simulink library "posAug_cl_old"  (R2022a)
settings: Solver=VariableStepAuto  StartTime=0.0  StopTime=10.0  RelTol=1e-3
undefined symbols (not defined in the file): aoaStart, elevSet, elevStart, env, FLIGHTCONTROLLER, fltCtrl, initializeBussesFromBlock, intSat, pathLaps, pathLapsYaw, posAug, rollAmp, rollFreq, rollPhase, sEstim, slfExitTime, thetaIGain, thetaPGain, vhcl, yawAmp, yawFreq, yawPhase
libraries: slpidlib x10, simulink x5, posAug_cl_new x4, velocityAngle_ul x4, dspsigops x3, pathFollowingCtrlAoATurb_cl x1, pathFollowingCtrlAoATurbCoef_cl x1, courseFollowLookAhead_cl x1, ctrlAllocMatrix3CompCoef_cl x1, eulAng2RotMat_ul x1, $bdroot x1, angleBtw2Vecs_ul x1
(part 2 of 3)

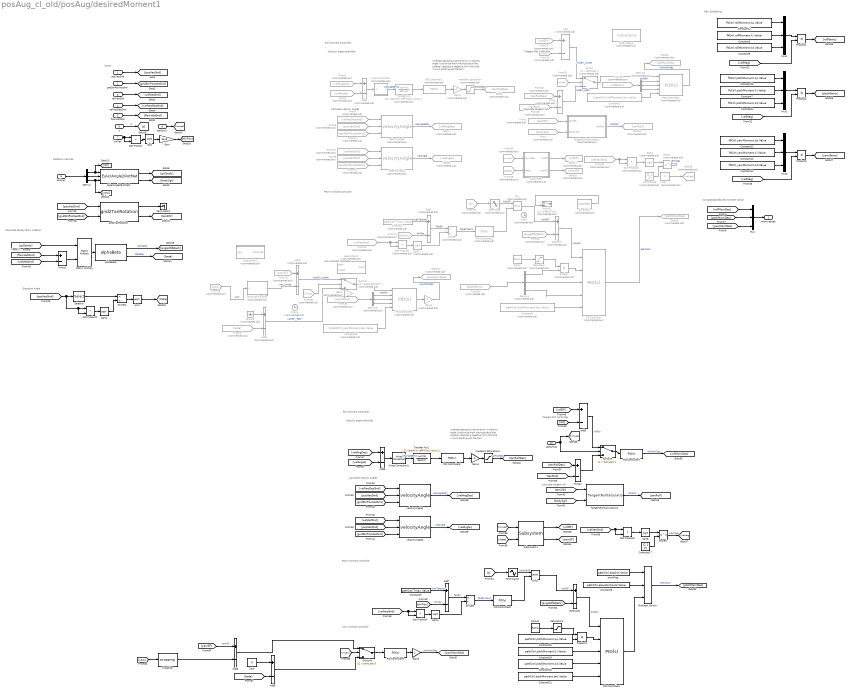
== system posAug_cl_old/posAug/desiredMoment1 ==
  note: Elevation Angle
  note: Yaw moment controller
  note: Pitch moment controller
  note: Inverted because a potive error
      | in velocity angle (clockwise from the
      | outside of the sphere) requires a negative
      | roll (With the X-Axis pointing out the tail)
  note: Velocity angle controller
  note: Inputs
  note: Rotation matrices
  note: Calculate velocity angles
  note: Calculate tangent roll
  note: Tangent Roll Controller
  note: Concatenate desired moment vector
  note: Calculate aerodynamic sideslip
  note: Roll Moment Controller
  note: Gain Scheduling
  note: Inverted because a potive error
      | in velocity angle (clockwise from the
      | outside of the sphere) requires a negative
      | roll (With the X-Axis pointing out the tail)
  note: Velocity angle controller
  note: Calculate tangent roll
  note: Calculate velocity angles
  note: Yaw moment controller
  note: Pitch moment controller
  note: Tangent Roll Controller
  note: Roll Moment Controller
  posVecGnd : Inport
  gndStnPosVecGnd : Inport  Port=2
  velVecGnd : Inport  Port=3
  velVecDesGnd : Inport  Port=4
  flowVecGnd : Inport  Port=5
  eulAng : Inport  Port=6
  thrTen : Inport  Port=7
  s : Inport  Port=8
  lapNumS : Inport  Port=9
  lapNumS1 : Inport  Port=10
  Add{,1..4} (5 alike) : Sum  Commented=on  Inputs=+-
  Add{5..9} (5 alike) : Sum  Inputs=+-
  Asin : Trigonometry  Operator=asin
  Clock : Clock  Commented=on
  Clock1 : Clock  Commented=on
  Constant : Constant  Commented=on  Value=pathCtrl.Tmax.Value
  Constant1 : Constant  Commented=on  Value=aoaStart
  Constant10 : Constant  Value=fltCtrl.yawMoment.ki.Value
  Constant11 : Constant  Value=fltCtrl.yawMoment.kd.Value
  Constant12 : Constant  Value=fltCtrl.yawMoment.kp.Value
  Constant13 : Constant  Value=fltCtrl.pitchMoment.kp.Value
  Constant14 : Constant  Value=fltCtrl.rollMoment.kp.Value
  Constant15 : Constant  Commented=on  Value=[2 2 2]
  Constant16 : Constant  Commented=on  Value=1/pathCtrl.yawMoment.tau.Value
  Constant17 : Constant  Value=[2 2 2]
  Constant19 : Constant  Value=pathCtrl.pitchMoment.ki.Value
  Constant2 : Constant  Commented=on  Value=1/pathCtrl.rollMoment.tau.Value
  Constant20 : Constant  Value=pathCtrl.pitchMoment.kd.Value
  Constant21 : Constant  Value=pathCtrl.pitchMoment.tau.Value
  Constant22 : Constant  Value=pathCtrl.pitchMoment.kp.Value
  Constant3 : Constant  Value=pathCtrl.Tmax.Value
  Constant4 : Constant  Commented=on  Value=pathCtrl.pitchMoment.tau.Value
  Constant5 : Constant  Value=fltCtrl.rollMoment.ki.Value
  Constant6 : Constant  Value=pathCtrl.elevatorConst.Value
  Constant7 : Constant  Value=fltCtrl.pitchMoment.ki.Value
  Constant8 : Constant  Value=fltCtrl.pitchMoment.kd.Value
  Constant9 : Constant  Value=fltCtrl.rollMoment.kd.Value
  Demux : Demux  Outputs=3
  Demux1 : Demux  Commented=on  Outputs=3
  Demux2 : Demux  Commented=on  Outputs=3
  Demux3 : Demux  Commented=on  Outputs=3
  Divide : Product  Commented=on  Inputs=*/
  Divide1 : Product  Inputs=*/
  Divide2 : Product  Inputs=*/
  Dot Product{,2,4,6} (4 alike) : DotProduct  OutDataTypeStr=Inherit: Inherit via internal rule
  Dot Product1 : DotProduct  Commented=on  OutDataTypeStr=Inherit: Inherit via internal rule
  Dot Product3 : DotProduct  Commented=on  OutDataTypeStr=Inherit: Inherit via internal rule
  EulerAngle2RotMat1 : eulAng2RotMat_ul/EulerAngle2RotMat  SystemSampleTime=-1  VariantActivationTime=update diagram  Latency=0  AutoFrameSizeCalculation=off
  From : From  Commented=on  GotoTag=body2gr
  From1 : From  Commented=on  GotoTag=tan2Gr
  From10 : From  Commented=on  GotoTag=gndStnPosVecGnd
  From11 : From  Commented=on  GotoTag=gndStnPosVecGnd
  From12 : From  Commented=on  GotoTag=velVecGnd
  From13 : From  Commented=on  GotoTag=yawSP
  From14 : From  Commented=on  GotoTag=rollSP
  From19 : From  Commented=on  GotoTag=yaw
  From2 : From  Commented=on  GotoTag=velAngDes
  From20 : From  Commented=on  GotoTag=velVecGnd
  From21 : From  Commented=on  GotoTag=thrTen
  From22 : From  Commented=on  GotoTag=angleOfAttack
  From23 : From  Commented=on  GotoTag=s
  From24 : From  Commented=on  GotoTag=roll
  From26 : From  Commented=on  GotoTag=tanRollDes
  From28 : From  Commented=on  GotoTag=tanRoll
  From29 : From  Commented=on  GotoTag=theta
  From3 : From  Commented=on  GotoTag=velAngle
  From30 : From  Commented=on  GotoTag=lumLap
  From34 : From  Commented=on  GotoTag=velVecGnd
  From35 : From  Commented=on  GotoTag=lumLap
  From36 : From  Commented=on  GotoTag=lumLap
  From37 : From  Commented=on  GotoTag=beta
  From38 : From  Commented=on  GotoTag=yawGains
  From39 : From  Commented=on  GotoTag=pitchGains
  From40 : From  Commented=on  GotoTag=rollGains
  From7 : From  Commented=on  GotoTag=velVecDesGnd
  From8 : From  Commented=on  GotoTag=posVecGnd
  From9 : From  Commented=on  GotoTag=posVecGnd
  Gain : Gain  Gain=1e-3
  Gain1 : Gain  Commented=on  Gain=-1
  Gain2 : Gain  Commented=on
  Gain3 : Gain  Commented=on
  Gain4 : Gain  Gain=-1
  Gain5 : Gain
  Goto10 : Goto  Commented=on  GotoTag=tanRoll
  Goto12 : Goto  Commented=on  GotoTag=rollMomDes
  Goto13 : Goto  Commented=on  GotoTag=yawMomDes
  Goto15 : Goto  Commented=on  GotoTag=pitchMomDes
  Goto17 : Goto  Commented=on  GotoTag=rollSP
  Goto20 : Goto  Commented=on  GotoTag=yawSP
  Goto28 : Goto  Commented=on  GotoTag=velMag
  Goto7 : Goto  Commented=on  GotoTag=velAngDes
  Goto8 : Goto  Commented=on  GotoTag=velAngle
  Goto9 : Goto  Commented=on  GotoTag=tanRollDes
  Ground : Ground  Commented=on
  MATLAB Function : MATLAB Function  Commented=on  TreatAsAtomicUnit=on
  Matrix Multiply : Product  Multiplication=Matrix(*)
  Min : MinMax  Commented=on  Inputs=2
  Min1 : MinMax  Inputs=2
  Minus : Sum  Commented=on  Inputs=+-
  Minus1 : Sum  Inputs=+-
  Minus2 : Sum  Inputs=+-
  Multiport Switch : MultiPortSwitch  DataPortOrder=Specify indices  Inputs=2  DataPortIndices={0,1}  SaturateOnIntegerOverflow=off  InputSameDT=off
  Mux{,1..3} (4 alike) : Mux  Inputs=3
  One : Constant  Commented=on  OutDataTypeStr=Inherit: Inherit via back propagation
  PID Controller : slpidlib/PID Controller  Commented=on  Controller=PID  Form=Parallel  TimeDomain=Continuous-time  UseExternalTs=off  SampleTime=-1  IntegratorMethod=Forward Euler  FilterMethod=Forward Euler  ControllerParametersSource=external  P=pathCtrl.pitchMoment.kp.Value  I=pathCtrl.pitchMoment.ki.Value  UseKiTs=off  D=pathCtrl.pitchMoment.kd.Value  N=1/pathCtrl.pitchMoment.tau.Value  UseFilter=on  TunerSelectOption=Transfer Function Based (PID Tuner App)  InitialConditionSource=internal  InitialConditionForIntegrator=0  InitialConditionForFilter=0  DifferentiatorICPrevScaledInput=0  ExternalReset=none  TrackingMode=off  Kt=1  LimitOutput=off  SatLimitsSource=internal  UpperSaturationLimit=inf  LowerSaturationLimit=-100  LinearizeAsGain=on  AntiWindupMode=clamping  Kb=1  POutMin=[]  POutMax=[]  IOutMin=[]  IOutMax=[]  DOutMin=[]  DOutMax=[]  NOutMin=[]  NOutMax=[]  SumOutMin=[]  SumOutMax=[]  SaturationOutMin=[]  SaturationOutMax=[]  PParamMin=[]  PParamMax=[]  IParamMin=[]  IParamMax=[]  DParamMin=[]  DParamMax=[]  NParamMin=[]  NParamMax=[]  KbParamMin=[]  KbParamMax=[]  KtParamMin=[]  KtParamMax=[]  KbOutMin=[]  KbOutMax=[]  KtOutMin=[]  KtOutMax=[]  IntegratorOutMin=[]  IntegratorOutMax=[]  FilterOutMin=[]  FilterOutMax=[]  SumI1OutMin=[]  SumI1OutMax=[]  SumI2OutMin=[]  SumI2OutMax=[]  SumI3OutMin=[]  SumI3OutMax=[]  SumI4OutMin=[]  SumI4OutMax=[]  SumDOutMin=[]  SumDOutMax=[]  DifferentiatorOutMin=[]  DifferentiatorOutMax=[]  FilterDiffOutCoefMin=[]  FilterDiffOutCoefMax=[]  ReciprocalOutMin=[]  ReciprocalOutMax=[]  SumDenOutMin=[]  SumDenOutMax=[]  SumNumOutMin=[]  SumNumOutMax=[]  DivideOutMin=[]  DivideOutMax=[]  UdiffTsProdOutMin=[]  UdiffTsProdOutMax=[]  NTsProdOutMin=[]  NTsProdOutMax=[]  UintegralTsProdOutMin=[]  UintegralTsProdOutMax=[]  UngainTsProdOutMin=[]  UngainTsProdOutMax=[]  IntegratorContinuousStateAttributes=''  IntegratorStateMustResolveToSignalObject=off  IntegratorRTWStateStorageClass=Auto  FilterContinuousStateAttributes=''  FilterStateMustResolveToSignalObject=off  FilterRTWStateStorageClass=Auto  ParallelPVariant=ExternalParameters  IdealPVariant=Disabled  IVariant=ExternalParameters  DVariant=ExternalParameters  IntegratorVariant=Continuous  SatVariant=Disabled  AWVariant=Passthrough  PCopyVariant=Disabled  TRVariant=Disabled  FdbkBlocksVariant=Forward  IdealPFdbkVariant=Disabled  SatFdbkVariant=Disabled  DerivativeFilterVariant=ContFilter  NVariant=ExternalParameters  NCopyVariant=Disabled  FilterICVariant=InternalICsFilter  IntegratorICVariant=InternalICs  ExternalResetVariant=Disabled  TRSumVariant=Passthrough  SumFdbkVariant=Disabled  SumVariant=Sum_PID  TsampFilterVariant=InternalTs  TsampNgainVariant=Passthrough  TsampIntegralVariant=Passthrough  ExternalSaturationOutDataTypeStr=Inherit: Same as second input  aMode=0
  PID Controller1 : slpidlib/PID Controller  Commented=on  Controller=PID  Form=Parallel  TimeDomain=Continuous-time  UseExternalTs=off  SampleTime=-1  IntegratorMethod=Forward Euler  FilterMethod=Forward Euler  ControllerParametersSource=internal  P=pathCtrl.tanRoll.kp.Value  I=pathCtrl.tanRoll.ki.Value  UseKiTs=off  D=pathCtrl.tanRoll.kd.Value  N=1/pathCtrl.tanRoll.tau.Value  UseFilter=on  TunerSelectOption=Transfer Function Based (PID Tuner App)  InitialConditionSource=internal  InitialConditionForIntegrator=0  InitialConditionForFilter=0  DifferentiatorICPrevScaledInput=0  ExternalReset=none  TrackingMode=off  Kt=1  LimitOutput=off  SatLimitsSource=internal  UpperSaturationLimit=inf  LowerSaturationLimit=-100  LinearizeAsGain=on  AntiWindupMode=clamping  Kb=1  POutMin=[]  POutMax=[]  IOutMin=[]  IOutMax=[]  DOutMin=[]  DOutMax=[]  NOutMin=[]  NOutMax=[]  SumOutMin=[]  SumOutMax=[]  SaturationOutMin=[]  SaturationOutMax=[]  PParamMin=[]  PParamMax=[]  IParamMin=[]  IParamMax=[]  DParamMin=[]  DParamMax=[]  NParamMin=[]  NParamMax=[]  KbParamMin=[]  KbParamMax=[]  KtParamMin=[]  KtParamMax=[]  KbOutMin=[]  KbOutMax=[]  KtOutMin=[]  KtOutMax=[]  IntegratorOutMin=[]  IntegratorOutMax=[]  FilterOutMin=[]  FilterOutMax=[]  SumI1OutMin=[]  SumI1OutMax=[]  SumI2OutMin=[]  SumI2OutMax=[]  SumI3OutMin=[]  SumI3OutMax=[]  SumI4OutMin=[]  SumI4OutMax=[]  SumDOutMin=[]  SumDOutMax=[]  DifferentiatorOutMin=[]  DifferentiatorOutMax=[]  FilterDiffOutCoefMin=[]  FilterDiffOutCoefMax=[]  ReciprocalOutMin=[]  ReciprocalOutMax=[]  SumDenOutMin=[]  SumDenOutMax=[]  SumNumOutMin=[]  SumNumOutMax=[]  DivideOutMin=[]  DivideOutMax=[]  UdiffTsProdOutMin=[]  UdiffTsProdOutMax=[]  NTsProdOutMin=[]  NTsProdOutMax=[]  UintegralTsProdOutMin=[]  UintegralTsProdOutMax=[]  UngainTsProdOutMin=[]  UngainTsProdOutMax=[]  IntegratorContinuousStateAttributes=''  IntegratorStateMustResolveToSignalObject=off  IntegratorRTWStateStorageClass=Auto  FilterContinuousStateAttributes=''  FilterStateMustResolveToSignalObject=off  FilterRTWStateStorageClass=Auto  ParallelPVariant=InternalParameters  IdealPVariant=Disabled  IVariant=InternalParameters  DVariant=InternalParameters  IntegratorVariant=Continuous  SatVariant=Disabled  AWVariant=Passthrough  PCopyVariant=Disabled  TRVariant=Disabled  FdbkBlocksVariant=Forward  IdealPFdbkVariant=Disabled  SatFdbkVariant=Disabled  DerivativeFilterVariant=ContFilter  NVariant=InternalParameters  NCopyVariant=Disabled  FilterICVariant=InternalICsFilter  IntegratorICVariant=InternalICs  ExternalResetVariant=Disabled  TRSumVariant=Passthrough  SumFdbkVariant=Disabled  SumVariant=Sum_PID  TsampFilterVariant=InternalTs  TsampNgainVariant=Passthrough  TsampIntegralVariant=Passthrough  ExternalSaturationOutDataTypeStr=Inherit: Same as second input  aMode=0
  PID Controller2 : slpidlib/PID Controller  Commented=on  Controller=PID  Form=Parallel  TimeDomain=Continuous-time  UseExternalTs=off  SampleTime=-1  IntegratorMethod=Forward Euler  FilterMethod=Forward Euler  ControllerParametersSource=external  P=pathCtrl.pitchMoment.kp.Value  I=pathCtrl.pitchMoment.ki.Value  UseKiTs=off  D=pathCtrl.pitchMoment.kd.Value  N=1/pathCtrl.pitchMoment.tau.Value  UseFilter=on  TunerSelectOption=Transfer Function Based (PID Tuner App)  InitialConditionSource=internal  InitialConditionForIntegrator=0  InitialConditionForFilter=0  DifferentiatorICPrevScaledInput=0  ExternalReset=none  TrackingMode=off  Kt=1  LimitOutput=off  SatLimitsSource=internal  UpperSaturationLimit=inf  LowerSaturationLimit=-100  LinearizeAsGain=on  AntiWindupMode=clamping  Kb=1  POutMin=[]  POutMax=[]  IOutMin=[]  IOutMax=[]  DOutMin=[]  DOutMax=[]  NOutMin=[]  NOutMax=[]  SumOutMin=[]  SumOutMax=[]  SaturationOutMin=[]  SaturationOutMax=[]  PParamMin=[]  PParamMax=[]  IParamMin=[]  IParamMax=[]  DParamMin=[]  DParamMax=[]  NParamMin=[]  NParamMax=[]  KbParamMin=[]  KbParamMax=[]  KtParamMin=[]  KtParamMax=[]  KbOutMin=[]  KbOutMax=[]  KtOutMin=[]  KtOutMax=[]  IntegratorOutMin=[]  IntegratorOutMax=[]  FilterOutMin=[]  FilterOutMax=[]  SumI1OutMin=[]  SumI1OutMax=[]  SumI2OutMin=[]  SumI2OutMax=[]  SumI3OutMin=[]  SumI3OutMax=[]  SumI4OutMin=[]  SumI4OutMax=[]  SumDOutMin=[]  SumDOutMax=[]  DifferentiatorOutMin=[]  DifferentiatorOutMax=[]  FilterDiffOutCoefMin=[]  FilterDiffOutCoefMax=[]  ReciprocalOutMin=[]  ReciprocalOutMax=[]  SumDenOutMin=[]  SumDenOutMax=[]  SumNumOutMin=[]  SumNumOutMax=[]  DivideOutMin=[]  DivideOutMax=[]  UdiffTsProdOutMin=[]  UdiffTsProdOutMax=[]  NTsProdOutMin=[]  NTsProdOutMax=[]  UintegralTsProdOutMin=[]  UintegralTsProdOutMax=[]  UngainTsProdOutMin=[]  UngainTsProdOutMax=[]  IntegratorContinuousStateAttributes=''  IntegratorStateMustResolveToSignalObject=off  IntegratorRTWStateStorageClass=Auto  FilterContinuousStateAttributes=''  FilterStateMustResolveToSignalObject=off  FilterRTWStateStorageClass=Auto  ParallelPVariant=ExternalParameters  IdealPVariant=Disabled  IVariant=ExternalParameters  DVariant=ExternalParameters  IntegratorVariant=Continuous  SatVariant=Disabled  AWVariant=Passthrough  PCopyVariant=Disabled  TRVariant=Disabled  FdbkBlocksVariant=Forward  IdealPFdbkVariant=Disabled  SatFdbkVariant=Disabled  DerivativeFilterVariant=ContFilter  NVariant=ExternalParameters  NCopyVariant=Disabled  FilterICVariant=InternalICsFilter  IntegratorICVariant=InternalICs  ExternalResetVariant=Disabled  TRSumVariant=Passthrough  SumFdbkVariant=Disabled  SumVariant=Sum_PID  TsampFilterVariant=InternalTs  TsampNgainVariant=Passthrough  TsampIntegralVariant=Passthrough  ExternalSaturationOutDataTypeStr=Inherit: Same as second input  aMode=0
  PID Controller3 : slpidlib/PID Controller  Commented=on  Controller=PID  Form=Parallel  TimeDomain=Continuous-time  UseExternalTs=off  SampleTime=-1  IntegratorMethod=Forward Euler  FilterMethod=Forward Euler  ControllerParametersSource=internal  P=pathCtrl.alphaCtrl.kp.Value  I=pathCtrl.alphaCtrl.ki.Value  UseKiTs=off  D=pathCtrl.alphaCtrl.kd.Value  N=1/pathCtrl.alphaCtrl.tau.Value  UseFilter=on  TunerSelectOption=Transfer Function Based (PID Tuner App)  InitialConditionSource=internal  InitialConditionForIntegrator=0  InitialConditionForFilter=0  DifferentiatorICPrevScaledInput=0  ExternalReset=none  TrackingMode=off  Kt=1  LimitOutput=on  SatLimitsSource=internal  UpperSaturationLimit=pathCtrl.AoAConst.Value  LowerSaturationLimit=pathCtrl.AoAmin.Value  LinearizeAsGain=on  AntiWindupMode=clamping  Kb=1  POutMin=[]  POutMax=[]  IOutMin=[]  IOutMax=[]  DOutMin=[]  DOutMax=[]  NOutMin=[]  NOutMax=[]  SumOutMin=[]  SumOutMax=[]  SaturationOutMin=[]  SaturationOutMax=[]  PParamMin=[]  PParamMax=[]  IParamMin=[]  IParamMax=[]  DParamMin=[]  DParamMax=[]  NParamMin=[]  NParamMax=[]  KbParamMin=[]  KbParamMax=[]  KtParamMin=[]  KtParamMax=[]  KbOutMin=[]  KbOutMax=[]  KtOutMin=[]  KtOutMax=[]  IntegratorOutMin=[]  IntegratorOutMax=[]  FilterOutMin=[]  FilterOutMax=[]  SumI1OutMin=[]  SumI1OutMax=[]  SumI2OutMin=[]  SumI2OutMax=[]  SumI3OutMin=[]  SumI3OutMax=[]  SumI4OutMin=[]  SumI4OutMax=[]  SumDOutMin=[]  SumDOutMax=[]  DifferentiatorOutMin=[]  DifferentiatorOutMax=[]  FilterDiffOutCoefMin=[]  FilterDiffOutCoefMax=[]  ReciprocalOutMin=[]  ReciprocalOutMax=[]  SumDenOutMin=[]  SumDenOutMax=[]  SumNumOutMin=[]  SumNumOutMax=[]  DivideOutMin=[]  DivideOutMax=[]  UdiffTsProdOutMin=[]  UdiffTsProdOutMax=[]  NTsProdOutMin=[]  NTsProdOutMax=[]  UintegralTsProdOutMin=[]  UintegralTsProdOutMax=[]  UngainTsProdOutMin=[]  UngainTsProdOutMax=[]  IntegratorContinuousStateAttributes=''  IntegratorStateMustResolveToSignalObject=off  IntegratorRTWStateStorageClass=Auto  FilterContinuousStateAttributes=''  FilterStateMustResolveToSignalObject=off  FilterRTWStateStorageClass=Auto  ParallelPVariant=InternalParameters  IdealPVariant=Disabled  IVariant=InternalParameters  DVariant=InternalParameters  IntegratorVariant=Continuous  SatVariant=Enabled  AWVariant=ContClampingParallel  PCopyVariant=Disabled  TRVariant=Disabled  FdbkBlocksVariant=Forward  IdealPFdbkVariant=Disabled  SatFdbkVariant=Disabled  DerivativeFilterVariant=ContFilter  NVariant=InternalParameters  NCopyVariant=Disabled  FilterICVariant=InternalICsFilter  IntegratorICVariant=InternalICs  ExternalResetVariant=Disabled  TRSumVariant=Passthrough  SumFdbkVariant=Disabled  SumVariant=Sum_PID  TsampFilterVariant=InternalTs  TsampNgainVariant=Passthrough  TsampIntegralVariant=Passthrough  ExternalSaturationOutDataTypeStr=Inherit: Same as second input  aMode=0
  PID Controller4 : slpidlib/PID Controller  Controller=PID  Form=Parallel  TimeDomain=Continuous-time  UseExternalTs=off  SampleTime=-1  IntegratorMethod=Forward Euler  FilterMethod=Forward Euler  ControllerParametersSource=external  P=pathCtrl.pitchMoment.kp.Value  I=pathCtrl.pitchMoment.ki.Value  UseKiTs=off  D=pathCtrl.pitchMoment.kd.Value  N=1/pathCtrl.pitchMoment.tau.Value  UseFilter=on  TunerSelectOption=Transfer Function Based (PID Tuner App)  InitialConditionSource=internal  InitialConditionForIntegrator=0  InitialConditionForFilter=0  DifferentiatorICPrevScaledInput=0  ExternalReset=none  TrackingMode=off  Kt=1  LimitOutput=off  SatLimitsSource=internal  UpperSaturationLimit=inf  LowerSaturationLimit=-100  LinearizeAsGain=on  AntiWindupMode=clamping  Kb=1  POutMin=[]  POutMax=[]  IOutMin=[]  IOutMax=[]  DOutMin=[]  DOutMax=[]  NOutMin=[]  NOutMax=[]  SumOutMin=[]  SumOutMax=[]  SaturationOutMin=[]  SaturationOutMax=[]  PParamMin=[]  PParamMax=[]  IParamMin=[]  IParamMax=[]  DParamMin=[]  DParamMax=[]  NParamMin=[]  NParamMax=[]  KbParamMin=[]  KbParamMax=[]  KtParamMin=[]  KtParamMax=[]  KbOutMin=[]  KbOutMax=[]  KtOutMin=[]  KtOutMax=[]  IntegratorOutMin=[]  IntegratorOutMax=[]  FilterOutMin=[]  FilterOutMax=[]  SumI1OutMin=[]  SumI1OutMax=[]  SumI2OutMin=[]  SumI2OutMax=[]  SumI3OutMin=[]  SumI3OutMax=[]  SumI4OutMin=[]  SumI4OutMax=[]  SumDOutMin=[]  SumDOutMax=[]  DifferentiatorOutMin=[]  DifferentiatorOutMax=[]  FilterDiffOutCoefMin=[]  FilterDiffOutCoefMax=[]  ReciprocalOutMin=[]  ReciprocalOutMax=[]  SumDenOutMin=[]  SumDenOutMax=[]  SumNumOutMin=[]  SumNumOutMax=[]  DivideOutMin=[]  DivideOutMax=[]  UdiffTsProdOutMin=[]  UdiffTsProdOutMax=[]  NTsProdOutMin=[]  NTsProdOutMax=[]  UintegralTsProdOutMin=[]  UintegralTsProdOutMax=[]  UngainTsProdOutMin=[]  UngainTsProdOutMax=[]  IntegratorContinuousStateAttributes=''  IntegratorStateMustResolveToSignalObject=off  IntegratorRTWStateStorageClass=Auto  FilterContinuousStateAttributes=''  FilterStateMustResolveToSignalObject=off  FilterRTWStateStorageClass=Auto  ParallelPVariant=ExternalParameters  IdealPVariant=Disabled  IVariant=ExternalParameters  DVariant=ExternalParameters  IntegratorVariant=Continuous  SatVariant=Disabled  AWVariant=Passthrough  PCopyVariant=Disabled  TRVariant=Disabled  FdbkBlocksVariant=Forward  IdealPFdbkVariant=Disabled  SatFdbkVariant=Disabled  DerivativeFilterVariant=ContFilter  NVariant=ExternalParameters  NCopyVariant=Disabled  FilterICVariant=InternalICsFilter  IntegratorICVariant=InternalICs  ExternalResetVariant=Disabled  TRSumVariant=Passthrough  SumFdbkVariant=Disabled  SumVariant=Sum_PID  TsampFilterVariant=InternalTs  TsampNgainVariant=Passthrough  TsampIntegralVariant=Passthrough  ExternalSaturationOutDataTypeStr=Inherit: Same as second input  aMode=0
  PID Controller5 : slpidlib/PID Controller  Commented=on  Controller=PID  Form=Parallel  TimeDomain=Continuous-time  UseExternalTs=off  SampleTime=-1  IntegratorMethod=Forward Euler  FilterMethod=Forward Euler  ControllerParametersSource=external  P=pathCtrl.pitchMoment.kp.Value  I=pathCtrl.pitchMoment.ki.Value  UseKiTs=off  D=pathCtrl.pitchMoment.kd.Value  N=1/pathCtrl.pitchMoment.tau.Value  UseFilter=on  TunerSelectOption=Transfer Function Based (PID Tuner App)  InitialConditionSource=internal  InitialConditionForIntegrator=0  InitialConditionForFilter=0  DifferentiatorICPrevScaledInput=0  ExternalReset=none  TrackingMode=off  Kt=1  LimitOutput=off  SatLimitsSource=internal  UpperSaturationLimit=inf  LowerSaturationLimit=-100  LinearizeAsGain=on  AntiWindupMode=clamping  Kb=1  POutMin=[]  POutMax=[]  IOutMin=[]  IOutMax=[]  DOutMin=[]  DOutMax=[]  NOutMin=[]  NOutMax=[]  SumOutMin=[]  SumOutMax=[]  SaturationOutMin=[]  SaturationOutMax=[]  PParamMin=[]  PParamMax=[]  IParamMin=[]  IParamMax=[]  DParamMin=[]  DParamMax=[]  NParamMin=[]  NParamMax=[]  KbParamMin=[]  KbParamMax=[]  KtParamMin=[]  KtParamMax=[]  KbOutMin=[]  KbOutMax=[]  KtOutMin=[]  KtOutMax=[]  IntegratorOutMin=[]  IntegratorOutMax=[]  FilterOutMin=[]  FilterOutMax=[]  SumI1OutMin=[]  SumI1OutMax=[]  SumI2OutMin=[]  SumI2OutMax=[]  SumI3OutMin=[]  SumI3OutMax=[]  SumI4OutMin=[]  SumI4OutMax=[]  SumDOutMin=[]  SumDOutMax=[]  DifferentiatorOutMin=[]  DifferentiatorOutMax=[]  FilterDiffOutCoefMin=[]  FilterDiffOutCoefMax=[]  ReciprocalOutMin=[]  ReciprocalOutMax=[]  SumDenOutMin=[]  SumDenOutMax=[]  SumNumOutMin=[]  SumNumOutMax=[]  DivideOutMin=[]  DivideOutMax=[]  UdiffTsProdOutMin=[]  UdiffTsProdOutMax=[]  NTsProdOutMin=[]  NTsProdOutMax=[]  UintegralTsProdOutMin=[]  UintegralTsProdOutMax=[]  UngainTsProdOutMin=[]  UngainTsProdOutMax=[]  IntegratorContinuousStateAttributes=''  IntegratorStateMustResolveToSignalObject=off  IntegratorRTWStateStorageClass=Auto  FilterContinuousStateAttributes=''  FilterStateMustResolveToSignalObject=off  FilterRTWStateStorageClass=Auto  ParallelPVariant=ExternalParameters  IdealPVariant=Disabled  IVariant=ExternalParameters  DVariant=ExternalParameters  IntegratorVariant=Continuous  SatVariant=Disabled  AWVariant=Passthrough  PCopyVariant=Disabled  TRVariant=Disabled  FdbkBlocksVariant=Forward  IdealPFdbkVariant=Disabled  SatFdbkVariant=Disabled  DerivativeFilterVariant=ContFilter  NVariant=ExternalParameters  NCopyVariant=Disabled  FilterICVariant=InternalICsFilter  IntegratorICVariant=InternalICs  ExternalResetVariant=Disabled  TRSumVariant=Passthrough  SumFdbkVariant=Disabled  SumVariant=Sum_PID  TsampFilterVariant=InternalTs  TsampNgainVariant=Passthrough  TsampIntegralVariant=Passthrough  ExternalSaturationOutDataTypeStr=Inherit: Same as second input  aMode=0
  PID Controller6 : slpidlib/PID Controller  Controller=PID  Form=Parallel  TimeDomain=Continuous-time  UseExternalTs=off  SampleTime=-1  IntegratorMethod=Forward Euler  FilterMethod=Forward Euler  ControllerParametersSource=internal  P=pathCtrl.tanRoll.kp.Value  I=pathCtrl.tanRoll.ki.Value  UseKiTs=off  D=pathCtrl.tanRoll.kd.Value  N=1/pathCtrl.tanRoll.tau.Value  UseFilter=on  TunerSelectOption=Transfer Function Based (PID Tuner App)  InitialConditionSource=internal  InitialConditionForIntegrator=0  InitialConditionForFilter=0  DifferentiatorICPrevScaledInput=0  ExternalReset=none  TrackingMode=off  Kt=1  LimitOutput=off  SatLimitsSource=internal  UpperSaturationLimit=inf  LowerSaturationLimit=-100  LinearizeAsGain=on  AntiWindupMode=clamping  Kb=1  POutMin=[]  POutMax=[]  IOutMin=[]  IOutMax=[]  DOutMin=[]  DOutMax=[]  NOutMin=[]  NOutMax=[]  SumOutMin=[]  SumOutMax=[]  SaturationOutMin=[]  SaturationOutMax=[]  PParamMin=[]  PParamMax=[]  IParamMin=[]  IParamMax=[]  DParamMin=[]  DParamMax=[]  NParamMin=[]  NParamMax=[]  KbParamMin=[]  KbParamMax=[]  KtParamMin=[]  KtParamMax=[]  KbOutMin=[]  KbOutMax=[]  KtOutMin=[]  KtOutMax=[]  IntegratorOutMin=[]  IntegratorOutMax=[]  FilterOutMin=[]  FilterOutMax=[]  SumI1OutMin=[]  SumI1OutMax=[]  SumI2OutMin=[]  SumI2OutMax=[]  SumI3OutMin=[]  SumI3OutMax=[]  SumI4OutMin=[]  SumI4OutMax=[]  SumDOutMin=[]  SumDOutMax=[]  DifferentiatorOutMin=[]  DifferentiatorOutMax=[]  FilterDiffOutCoefMin=[]  FilterDiffOutCoefMax=[]  ReciprocalOutMin=[]  ReciprocalOutMax=[]  SumDenOutMin=[]  SumDenOutMax=[]  SumNumOutMin=[]  SumNumOutMax=[]  DivideOutMin=[]  DivideOutMax=[]  UdiffTsProdOutMin=[]  UdiffTsProdOutMax=[]  NTsProdOutMin=[]  NTsProdOutMax=[]  UintegralTsProdOutMin=[]  UintegralTsProdOutMax=[]  UngainTsProdOutMin=[]  UngainTsProdOutMax=[]  IntegratorContinuousStateAttributes=''  IntegratorStateMustResolveToSignalObject=off  IntegratorRTWStateStorageClass=Auto  FilterContinuousStateAttributes=''  FilterStateMustResolveToSignalObject=off  FilterRTWStateStorageClass=Auto  ParallelPVariant=InternalParameters  IdealPVariant=Disabled  IVariant=InternalParameters  DVariant=InternalParameters  IntegratorVariant=Continuous  SatVariant=Disabled  AWVariant=Passthrough  PCopyVariant=Disabled  TRVariant=Disabled  FdbkBlocksVariant=Forward  IdealPFdbkVariant=Disabled  SatFdbkVariant=Disabled  DerivativeFilterVariant=ContFilter  NVariant=InternalParameters  NCopyVariant=Disabled  FilterICVariant=InternalICsFilter  IntegratorICVariant=InternalICs  ExternalResetVariant=Disabled  TRSumVariant=Passthrough  SumFdbkVariant=Disabled  SumVariant=Sum_PID  TsampFilterVariant=InternalTs  TsampNgainVariant=Passthrough  TsampIntegralVariant=Passthrough  ExternalSaturationOutDataTypeStr=Inherit: Same as second input  aMode=0
  PID Controller7 : slpidlib/PID Controller  Controller=PID  Form=Parallel  TimeDomain=Continuous-time  UseExternalTs=off  SampleTime=-1  IntegratorMethod=Forward Euler  FilterMethod=Forward Euler  ControllerParametersSource=internal  P=pathCtrl.rollMoment.kp.Value  I=pathCtrl.rollMoment.ki.Value  UseKiTs=off  D=pathCtrl.rollMoment.kd.Value  N=1/pathCtrl.rollMoment.tau.Value  UseFilter=on  TunerSelectOption=Transfer Function Based (PID Tuner App)  InitialConditionSource=internal  InitialConditionForIntegrator=0  InitialConditionForFilter=0  DifferentiatorICPrevScaledInput=0  ExternalReset=none  TrackingMode=off  Kt=1  LimitOutput=off  SatLimitsSource=internal  UpperSaturationLimit=inf  LowerSaturationLimit=-100  LinearizeAsGain=on  AntiWindupMode=clamping  Kb=1  POutMin=[]  POutMax=[]  IOutMin=[]  IOutMax=[]  DOutMin=[]  DOutMax=[]  NOutMin=[]  NOutMax=[]  SumOutMin=[]  SumOutMax=[]  SaturationOutMin=[]  SaturationOutMax=[]  PParamMin=[]  PParamMax=[]  IParamMin=[]  IParamMax=[]  DParamMin=[]  DParamMax=[]  NParamMin=[]  NParamMax=[]  KbParamMin=[]  KbParamMax=[]  KtParamMin=[]  KtParamMax=[]  KbOutMin=[]  KbOutMax=[]  KtOutMin=[]  KtOutMax=[]  IntegratorOutMin=[]  IntegratorOutMax=[]  FilterOutMin=[]  FilterOutMax=[]  SumI1OutMin=[]  SumI1OutMax=[]  SumI2OutMin=[]  SumI2OutMax=[]  SumI3OutMin=[]  SumI3OutMax=[]  SumI4OutMin=[]  SumI4OutMax=[]  SumDOutMin=[]  SumDOutMax=[]  DifferentiatorOutMin=[]  DifferentiatorOutMax=[]  FilterDiffOutCoefMin=[]  FilterDiffOutCoefMax=[]  ReciprocalOutMin=[]  ReciprocalOutMax=[]  SumDenOutMin=[]  SumDenOutMax=[]  SumNumOutMin=[]  SumNumOutMax=[]  DivideOutMin=[]  DivideOutMax=[]  UdiffTsProdOutMin=[]  UdiffTsProdOutMax=[]  NTsProdOutMin=[]  NTsProdOutMax=[]  UintegralTsProdOutMin=[]  UintegralTsProdOutMax=[]  UngainTsProdOutMin=[]  UngainTsProdOutMax=[]  IntegratorContinuousStateAttributes=''  IntegratorStateMustResolveToSignalObject=off  IntegratorRTWStateStorageClass=Auto  FilterContinuousStateAttributes=''  FilterStateMustResolveToSignalObject=off  FilterRTWStateStorageClass=Auto  ParallelPVariant=InternalParameters  IdealPVariant=Disabled  IVariant=InternalParameters  DVariant=InternalParameters  IntegratorVariant=Continuous  SatVariant=Disabled  AWVariant=Passthrough  PCopyVariant=Disabled  TRVariant=Disabled  FdbkBlocksVariant=Forward  IdealPFdbkVariant=Disabled  SatFdbkVariant=Disabled  DerivativeFilterVariant=ContFilter  NVariant=InternalParameters  NCopyVariant=Disabled  FilterICVariant=InternalICsFilter  IntegratorICVariant=InternalICs  ExternalResetVariant=Disabled  TRSumVariant=Passthrough  SumFdbkVariant=Disabled  SumVariant=Sum_PID  TsampFilterVariant=InternalTs  TsampNgainVariant=Passthrough  TsampIntegralVariant=Passthrough  ExternalSaturationOutDataTypeStr=Inherit: Same as second input  aMode=0
  PID Controller8 : slpidlib/PID Controller  Controller=PID  Form=Parallel  TimeDomain=Continuous-time  UseExternalTs=off  SampleTime=-1  IntegratorMethod=Forward Euler  FilterMethod=Forward Euler  ControllerParametersSource=internal  P=pathCtrl.alphaCtrl.kp.Value  I=pathCtrl.alphaCtrl.ki.Value  UseKiTs=off  D=pathCtrl.alphaCtrl.kd.Value  N=1/pathCtrl.alphaCtrl.tau.Value  UseFilter=on  TunerSelectOption=Transfer Function Based (PID Tuner App)  InitialConditionSource=internal  InitialConditionForIntegrator=0  InitialConditionForFilter=0  DifferentiatorICPrevScaledInput=0  ExternalReset=none  TrackingMode=off  Kt=1  LimitOutput=on  SatLimitsSource=internal  UpperSaturationLimit=pathCtrl.AoAConst.Value  LowerSaturationLimit=pathCtrl.AoAmin.Value  LinearizeAsGain=on  AntiWindupMode=clamping  Kb=1  POutMin=[]  POutMax=[]  IOutMin=[]  IOutMax=[]  DOutMin=[]  DOutMax=[]  NOutMin=[]  NOutMax=[]  SumOutMin=[]  SumOutMax=[]  SaturationOutMin=[]  SaturationOutMax=[]  PParamMin=[]  PParamMax=[]  IParamMin=[]  IParamMax=[]  DParamMin=[]  DParamMax=[]  NParamMin=[]  NParamMax=[]  KbParamMin=[]  KbParamMax=[]  KtParamMin=[]  KtParamMax=[]  KbOutMin=[]  KbOutMax=[]  KtOutMin=[]  KtOutMax=[]  IntegratorOutMin=[]  IntegratorOutMax=[]  FilterOutMin=[]  FilterOutMax=[]  SumI1OutMin=[]  SumI1OutMax=[]  SumI2OutMin=[]  SumI2OutMax=[]  SumI3OutMin=[]  SumI3OutMax=[]  SumI4OutMin=[]  SumI4OutMax=[]  SumDOutMin=[]  SumDOutMax=[]  DifferentiatorOutMin=[]  DifferentiatorOutMax=[]  FilterDiffOutCoefMin=[]  FilterDiffOutCoefMax=[]  ReciprocalOutMin=[]  ReciprocalOutMax=[]  SumDenOutMin=[]  SumDenOutMax=[]  SumNumOutMin=[]  SumNumOutMax=[]  DivideOutMin=[]  DivideOutMax=[]  UdiffTsProdOutMin=[]  UdiffTsProdOutMax=[]  NTsProdOutMin=[]  NTsProdOutMax=[]  UintegralTsProdOutMin=[]  UintegralTsProdOutMax=[]  UngainTsProdOutMin=[]  UngainTsProdOutMax=[]  IntegratorContinuousStateAttributes=''  IntegratorStateMustResolveToSignalObject=off  IntegratorRTWStateStorageClass=Auto  FilterContinuousStateAttributes=''  FilterStateMustResolveToSignalObject=off  FilterRTWStateStorageClass=Auto  ParallelPVariant=InternalParameters  IdealPVariant=Disabled  IVariant=InternalParameters  DVariant=InternalParameters  IntegratorVariant=Continuous  SatVariant=Enabled  AWVariant=ContClampingParallel  PCopyVariant=Disabled  TRVariant=Disabled  FdbkBlocksVariant=Forward  IdealPFdbkVariant=Disabled  SatFdbkVariant=Disabled  DerivativeFilterVariant=ContFilter  NVariant=InternalParameters  NCopyVariant=Disabled  FilterICVariant=InternalICsFilter  IntegratorICVariant=InternalICs  ExternalResetVariant=Disabled  TRSumVariant=Passthrough  SumFdbkVariant=Disabled  SumVariant=Sum_PID  TsampFilterVariant=InternalTs  TsampNgainVariant=Passthrough  TsampIntegralVariant=Passthrough  ExternalSaturationOutDataTypeStr=Inherit: Same as second input  aMode=0
  PID Controller9 : slpidlib/PID Controller  Controller=PID  Form=Parallel  TimeDomain=Continuous-time  UseExternalTs=off  SampleTime=-1  IntegratorMethod=Forward Euler  FilterMethod=Forward Euler  ControllerParametersSource=internal  P=pathCtrl.yawMoment.kp.Value  I=pathCtrl.yawMoment.ki.Value  UseKiTs=off  D=pathCtrl.yawMoment.kd.Value  N=1/pathCtrl.yawMoment.tau.Value  UseFilter=on  TunerSelectOption=Transfer Function Based (PID Tuner App)  InitialConditionSource=internal  InitialConditionForIntegrator=0  InitialConditionForFilter=0  DifferentiatorICPrevScaledInput=0  ExternalReset=none  TrackingMode=off  Kt=1  LimitOutput=off  SatLimitsSource=internal  UpperSaturationLimit=inf  LowerSaturationLimit=-100  LinearizeAsGain=on  AntiWindupMode=clamping  Kb=1  POutMin=[]  POutMax=[]  IOutMin=[]  IOutMax=[]  DOutMin=[]  DOutMax=[]  NOutMin=[]  NOutMax=[]  SumOutMin=[]  SumOutMax=[]  SaturationOutMin=[]  SaturationOutMax=[]  PParamMin=[]  PParamMax=[]  IParamMin=[]  IParamMax=[]  DParamMin=[]  DParamMax=[]  NParamMin=[]  NParamMax=[]  KbParamMin=[]  KbParamMax=[]  KtParamMin=[]  KtParamMax=[]  KbOutMin=[]  KbOutMax=[]  KtOutMin=[]  KtOutMax=[]  IntegratorOutMin=[]  IntegratorOutMax=[]  FilterOutMin=[]  FilterOutMax=[]  SumI1OutMin=[]  SumI1OutMax=[]  SumI2OutMin=[]  SumI2OutMax=[]  SumI3OutMin=[]  SumI3OutMax=[]  SumI4OutMin=[]  SumI4OutMax=[]  SumDOutMin=[]  SumDOutMax=[]  DifferentiatorOutMin=[]  DifferentiatorOutMax=[]  FilterDiffOutCoefMin=[]  FilterDiffOutCoefMax=[]  ReciprocalOutMin=[]  ReciprocalOutMax=[]  SumDenOutMin=[]  SumDenOutMax=[]  SumNumOutMin=[]  SumNumOutMax=[]  DivideOutMin=[]  DivideOutMax=[]  UdiffTsProdOutMin=[]  UdiffTsProdOutMax=[]  NTsProdOutMin=[]  NTsProdOutMax=[]  UintegralTsProdOutMin=[]  UintegralTsProdOutMax=[]  UngainTsProdOutMin=[]  UngainTsProdOutMax=[]  IntegratorContinuousStateAttributes=''  IntegratorStateMustResolveToSignalObject=off  IntegratorRTWStateStorageClass=Auto  FilterContinuousStateAttributes=''  FilterStateMustResolveToSignalObject=off  FilterRTWStateStorageClass=Auto  ParallelPVariant=InternalParameters  IdealPVariant=Disabled  IVariant=InternalParameters  DVariant=InternalParameters  IntegratorVariant=Continuous  SatVariant=Disabled  AWVariant=Passthrough  PCopyVariant=Disabled  TRVariant=Disabled  FdbkBlocksVariant=Forward  IdealPFdbkVariant=Disabled  SatFdbkVariant=Disabled  DerivativeFilterVariant=ContFilter  NVariant=InternalParameters  NCopyVariant=Disabled  FilterICVariant=InternalICsFilter  IntegratorICVariant=InternalICs  ExternalResetVariant=Disabled  TRSumVariant=Passthrough  SumFdbkVariant=Disabled  SumVariant=Sum_PID  TsampFilterVariant=InternalTs  TsampNgainVariant=Passthrough  TsampIntegralVariant=Passthrough  ExternalSaturationOutDataTypeStr=Inherit: Same as second input  aMode=0
  Power : Math  Commented=on  Operator=pow
  Power1 : Math  Operator=pow
  Product : Product  Commented=on
  Product{1..4} (4 alike) : Product
  Ramp : simulink/Sources/Ramp  Commented=on  slope=0.05  start=100  InitialOutput=0.2
  Ramp1 : simulink/Sources/Ramp  slope=0.05  start=100  InitialOutput=0.2
  Saturation : Saturate  Commented=on  UpperLimit=1  LowerLimit=0.2
  Saturation1 : Saturate  UpperLimit=1  LowerLimit=0.2
  Selector : Selector  InputPortWidth=3  IndexOptions=Index vector (dialog)  Indices=[3]  OutputSizes=1
  Sine Wave : Sin  Commented=on  TimeSource=Use external signal  Amplitude=0  Bias=fltCtrl.AoAConst.Value  Frequency=4*pi  Phase=pi/2  SampleTime=0
  Sine Wave1 : Sin  TimeSource=Use external signal  Amplitude=0  Bias=fltCtrl.AoAConst.Value  Frequency=4*pi  Phase=pi/2  SampleTime=0
  Sqrt{,2,4,6} (4 alike) : Sqrt
  Sqrt1 : Sqrt  Commented=on
  Sqrt3 : Sqrt  Commented=on
  Subsystem : Subsystem  Commented=on
  Subsystem1 : Subsystem  Commented=on
  Subsystem2 : Subsystem  Commented=on
  Subsystem3 : $bdroot/posAug/desiredMoment1/Subsystem2  Commented=on  SystemSampleTime=-1  VariantActivationTime=update diagram  Latency=0  AutoFrameSizeCalculation=off
  Subsystem4 : posAug_cl_new/posAug/desiredMoment1/Subsystem  SystemSampleTime=-1  VariantActivationTime=update diagram  Latency=0  AutoFrameSizeCalculation=off
  Subtract : Sum  Commented=on  Inputs=+-
  Subtract1 : Sum  Inputs=+-
  Switch : Switch  Commented=on  Criteria=u2 > Threshold  Threshold=pathLaps-1  SaturateOnIntegerOverflow=off  InputSameDT=off
  Switch1 : Switch  Commented=on  Criteria=u2 > Threshold  Threshold=pathLapsYaw-1  SaturateOnIntegerOverflow=off  InputSameDT=off
  Switch2 : Switch  Commented=on  Criteria=u2 > Threshold  Threshold=slfExitTime  SaturateOnIntegerOverflow=off  InputSameDT=off
  Switch3 : Switch  Criteria=u2 > Threshold  Threshold=pathLaps-1  SaturateOnIntegerOverflow=off  InputSameDT=off
  Switch4 : Switch  Criteria=u2 > Threshold  Threshold=pathLaps-3  SaturateOnIntegerOverflow=off  InputSameDT=off
  TangentRollCalculation : Subsystem  Commented=on
  TangentRollCalculation1 : posAug_cl_new/posAug/desiredMoment1/TangentRollCalculation  SystemSampleTime=-1  VariantActivationTime=update diagram  Latency=0  AutoFrameSizeCalculation=off
  Terminator1 : Terminator
  Transfer Fcn : TransferFcn  Commented=on  Denominator=[pathCtrl.refFiltTau.Value 1]
  Transfer Fcn1 : TransferFcn  Denominator=[pathCtrl.refFiltTau.Value 1]
  Wrap Correction : Subsystem  Commented=on
  Wrap Correction1 : posAug_cl_new/posAug/desiredMoment1/Wrap Correction  SystemSampleTime=-1  VariantActivationTime=update diagram  Latency=0  AutoFrameSizeCalculation=off
  Zero : Constant  Value=0  OutDataTypeStr=Inherit: Inherit via back propagation
  alphaBeta : alphaBeta_ul/alphaBeta  SystemSampleTime=-1  VariantActivationTime=update diagram  Latency=0  AutoFrameSizeCalculation=off
  gnd2TanRotation : gnd2TanRotation_ul/gnd2TanRotation  SystemSampleTime=-1  VariantActivationTime=update diagram  Latency=0  AutoFrameSizeCalculation=off
  maxBank Saturation : Saturate  Commented=on  UpperLimit=pathCtrl.maxBank.upperLimit.Value  LowerLimit=pathCtrl.maxBank.lowerLimit.Value
  maxBank Saturation1 : Saturate  UpperLimit=pathCtrl.maxBank.upperLimit.Value  LowerLimit=pathCtrl.maxBank.lowerLimit.Value
  pitchFlag : Constant  Value=pathCtrl.AoACtrl.Value
  velocityAngle : velocityAngle_ul/velocityAngle  Commented=on  SystemSampleTime=-1  VariantActivationTime=update diagram  Latency=0  AutoFrameSizeCalculation=off
  velocityAngle1 : velocityAngle_ul/velocityAngle  Commented=on  SystemSampleTime=-1  VariantActivationTime=update diagram  Latency=0  AutoFrameSizeCalculation=off
  velocityAngle2 : velocityAngle_ul/velocityAngle  SystemSampleTime=-1  VariantActivationTime=update diagram  Latency=0  AutoFrameSizeCalculation=off
  velocityAngle3 : velocityAngle_ul/velocityAngle  SystemSampleTime=-1  VariantActivationTime=update diagram  Latency=0  AutoFrameSizeCalculation=off
  wrapping : posAug_cl_new/posAug/desiredMoment1/wrapping  SystemSampleTime=-1  VariantActivationTime=update diagram  Latency=0  AutoFrameSizeCalculation=off
  momVecDes : Outport  VectorParamsAs1DForOutWhenUnconnected=off
  wires:
  PID Controller3/1 -> Min/2
  From23/1 -> Sine Wave/1
  s/1 -> [s]  "S"
  Saturation/1 -> Product/1
  Product/1 -> PID Controller/2
  Demux1/1 -> Product/2
  Ramp/1 -> Saturation/1
  Constant4/1 -> PID Controller/5
  Demux1/3 -> PID Controller/4
  Demux1/2 -> PID Controller/3
  Constant/1 -> Add2/1  "maxTension"
  Add2/1 -> Divide/1  "TenErr"
  From21/1 -> Add2/2  "thrTen"
  Transfer Fcn/1 -> PID Controller1/1
  Demux/3 -> [yaw], EulerAngle2RotMat1/3
  Dot Product1/1 -> Sqrt1/1
  From20/1 -> Dot Product1/1, Dot Product1/2
  Gain/1 -> [thrTen]
  Dot Product/1 -> Sqrt/1
  Sqrt/1 -> Gain/1
  thrTen/1 -> Dot Product/1, Dot Product/2
  Subtract/1 -> PID Controller/1  "AoAerr"
  From22/1 -> Subtract/2
  PID Controller/1 -> Goto15/1  "elevMom"
  [pitchMomDes] -> Mux/2
  PID Controller5/1 -> Gain3/1
  PID Controller1/1 -> Gain1/1
  [yawMomDes] -> Mux/3
  gnd2TanRotation/1 -> Terminator1/1
  gnd2TanRotation/2 -> [tan2Gr]
  [gndStnPosVecGnd] -> gnd2TanRotation/2
  [posVecGnd] -> gnd2TanRotation/1
  From14/1 -> Add/1
  From24/1 -> Add/2
  From12/1 -> velocityAngle1/1
  From11/1 -> velocityAngle1/3
  From10/1 -> velocityAngle/3
  From9/1 -> velocityAngle1/2
  From8/1 -> velocityAngle/2
  From7/1 -> velocityAngle/1
  From3/1 -> Add1/2
  From2/1 -> Add1/1
  velocityAngle1/1 -> Goto8/1  "velAngle"
  velocityAngle/1 -> Goto7/1  "velAngleDes"
  velVecDesGnd/1 -> [velVecDesGnd]
  gndStnPosVecGnd/1 -> [gndStnPosVecGnd]
  alphaBeta/1 -> [angleOfAttack]  "alphaBdy"
  alphaBeta/2 -> [beta]  "betaBdy"
  Matrix Multiply/1 -> alphaBeta/1
  [gr2body] -> Matrix Multiply/1
  From/1 -> TangentRollCalculation/2(bdy2Inert)
  EulerAngle2RotMat1/1 -> [gr2body]
  EulerAngle2RotMat1/2 -> [body2gr]
  Demux/2 -> EulerAngle2RotMat1/2
  eulAng/1 -> Demux/1
  [flowVecGnd] -> Minus1/1
  [velVecGnd] -> Minus1/2
  Minus1/1 -> Matrix Multiply/2
  TangentRollCalculation/1(tanRoll) -> Goto10/1  "tanRoll"
  From1/1 -> TangentRollCalculation/1(tan2Gr)
  flowVecGnd/1 -> [flowVecGnd]
  Add1/1 -> Wrap Correction/1(u)
  maxBank Saturation/1 -> Goto9/1  "tanRollDes"
  Gain1/1 -> maxBank Saturation/1
  velVecGnd/1 -> [velVecGnd]
  posVecGnd/1 -> [posVecGnd]
  Wrap Correction/1(y) -> Transfer Fcn/1  "velAngleError"
  [rollMomDes] -> Mux/1
  PID Controller2/1 -> Goto12/1  "rollMomDes"
  Subsystem/1(rollSP) -> Goto17/1
  Subsystem/2(yawSP) -> Goto20/1
  From13/1 -> Add3/1
  Demux/1 -> [roll], EulerAngle2RotMat1/1
  From26/1 -> Minus/1
  From28/1 -> Minus/2
  [posVecGnd] -> Dot Product2/2, Dot Product2/1, Selector/1
  Dot Product2/1 -> Sqrt2/1
  Selector/1 -> Divide1/1
  Sqrt2/1 -> Divide1/2
  Divide1/1 -> Asin/1
  Asin/1 -> [theta]
  From29/1 -> Subsystem/2(theta)
  From30/1 -> Subsystem/1(numLaps)
  lapNumS/1 -> [lumLap]
  Product3/1 -> [yawGains]
  [velMag] -> Product3/2
  Constant5/1 -> Mux1/2
  Constant9/1 -> Mux1/3
  [velMag] -> Product2/2
  Constant7/1 -> Mux2/2
  Mux1/1 -> Product1/1
  Mux2/1 -> Product2/1
  Constant10/1 -> Mux3/2
  [velMag] -> Product1/2
  Constant13/1 -> Mux2/1
  Constant11/1 -> Mux3/3
  Constant12/1 -> Mux3/1
  Mux3/1 -> Product3/1
  Product1/1 -> [rollGains]
  Constant14/1 -> Mux1/1
  Product2/1 -> [pitchGains]
  Constant8/1 -> Mux2/3
  Constant15/1 -> Power/2
  From34/1 -> Dot Product3/2, Dot Product3/1
  Sqrt3/1 -> Power/1
  Dot Product3/1 -> Sqrt3/1
  From35/1 -> Switch/2
  From36/1 -> Switch1/2
  From37/1 -> Add4/2
  Demux3/2 -> PID Controller5/3
  Demux3/1 -> PID Controller5/2
  Demux3/3 -> PID Controller5/4
  From38/1 -> Demux3/1
  Constant16/1 -> PID Controller5/5
  From39/1 -> Demux1/1
  From40/1 -> Demux2/1
  Demux2/1 -> PID Controller2/2
  Demux2/3 -> PID Controller2/4
  Demux2/2 -> PID Controller2/3
  Constant2/1 -> PID Controller2/5
  Power/1 -> ?  "velmags"
  Gain3/1 -> Goto13/1  "yawMomDes"
  Ground/1 -> Add4/1
  Mux/1 -> momVecDes/1
  Divide/1 -> PID Controller3/1  "TenErrNorm"
  Sqrt1/1 -> Divide/2
  Minus/1 -> Switch/3  "rollErr_path"
  Add/1 -> Switch/1  "rollErr_orient"
  Switch/1 -> PID Controller2/1  "rollErr"
  Constant1/1 -> Switch2/3
  Sine Wave/1 -> Min/1  "AoASP"
  Add4/1 -> Switch1/3  "yawErr_Path"
  Add3/1 -> Switch1/1  "yawErr_orient"
  Switch1/1 -> PID Controller5/1  "yawErr"
  From19/1 -> MATLAB Function/1(u)  "yaw"
  One/1 -> Goto28/1
  MATLAB Function/1(y) -> Add3/2  "yaw_Wrap"
  Min/1 -> Subtract/1  "AoASP"
  [velVecDesGnd] -> velocityAngle2/1
  Constant17/1 -> Power1/2
  Constant20/1 -> PID Controller4/4
  Subsystem4/2 -> [yawSP]
  PID Controller8/1 -> Min1/2
  Subsystem4/1 -> [rollSP]
  Wrap Correction1/1 -> Transfer Fcn1/1  "velAngleError"
  [s] -> Sine Wave1/1
  Add5/1 -> Switch3/1  "rollErr"
  [gndStnPosVecGnd] -> velocityAngle2/3
  Gain4/1 -> maxBank Saturation1/1
  [tan2Gr] -> TangentRollCalculation1/1
  maxBank Saturation1/1 -> [tanRollDes]  "tanRollDes"
  velocityAngle2/1 -> [velAngDes]  "velAngleDes"
  [angleOfAttack] -> Subtract1/2
  velocityAngle3/1 -> [velAngle]  "velAngle"
  [posVecGnd] -> velocityAngle3/2
  [velAngDes] -> Add6/1
  Constant22/1 -> Product4/2
  Minus2/1 -> Switch3/3
  Sqrt6/1 -> Power1/1
  Subtract1/1 -> PID Controller4/1  "AoAerr"
  [body2gr] -> TangentRollCalculation1/2
  Sqrt4/1 -> Divide2/2
  Power1/1 -> [velMag]  "velmags"
  PID Controller4/1 -> Multiport Switch/3
  Divide2/1 -> PID Controller8/1  "TenErrNorm"
  Sine Wave1/1 -> Min1/1  "varAoASP"
  Saturation1/1 -> Product4/1
  Add6/1 -> Wrap Correction1/1
  Switch3/1 -> PID Controller7/1
  Constant3/1 -> Add7/1  "maxTension"
  [rollSP] -> Add5/1
  [roll] -> Add5/2
  PID Controller7/1 -> [rollMomDes]  "rollMomDes"
  [theta] -> Subsystem4/2
  [tanRoll] -> Minus2/2
  [lumLap] -> Subsystem4/1
  lapNumS1/1 -> Switch3/2, [lumLap]
  [tanRollDes] -> Minus2/1
  [velVecGnd] -> Dot Product6/1, Dot Product6/2
  TangentRollCalculation1/1 -> [tanRoll]  "tanRoll"
  [posVecGnd] -> velocityAngle2/2
  Constant6/1 -> Multiport Switch/2
  PID Controller9/1 -> Gain5/1
  Multiport Switch/1 -> [pitchMomDes]  "elevMom"
  [gndStnPosVecGnd] -> velocityAngle3/3
  [velVecGnd] -> velocityAngle3/1
  Constant21/1 -> PID Controller4/5
  pitchFlag/1 -> Multiport Switch/1
  Dot Product6/1 -> Sqrt6/1
  Add7/1 -> Divide2/1  "TenErr"
  Transfer Fcn1/1 -> PID Controller6/1
  Gain5/1 -> [yawMomDes]  "yawMomDes"
  Dot Product4/1 -> Sqrt4/1
  Ramp1/1 -> Saturation1/1
  [thrTen] -> Add7/2  "thrTen"
  Constant19/1 -> PID Controller4/3
  PID Controller6/1 -> Gain4/1
  Min1/1 -> Subtract1/1  "AoASP"
  [velVecGnd] -> Dot Product4/1, Dot Product4/2
  Product4/1 -> PID Controller4/2
  Switch4/1 -> PID Controller9/1
  [velAngle] -> Add6/2
  wrapping/1 -> Add8/2
  Zero/1 -> Add9/1
  [yaw] -> wrapping/1
  [beta] -> Add9/2
  Add8/1 -> Switch4/1
  Add9/1 -> Switch4/3
  [yawSP] -> Add8/1  "yawSP"
  [lumLap] -> Switch4/2

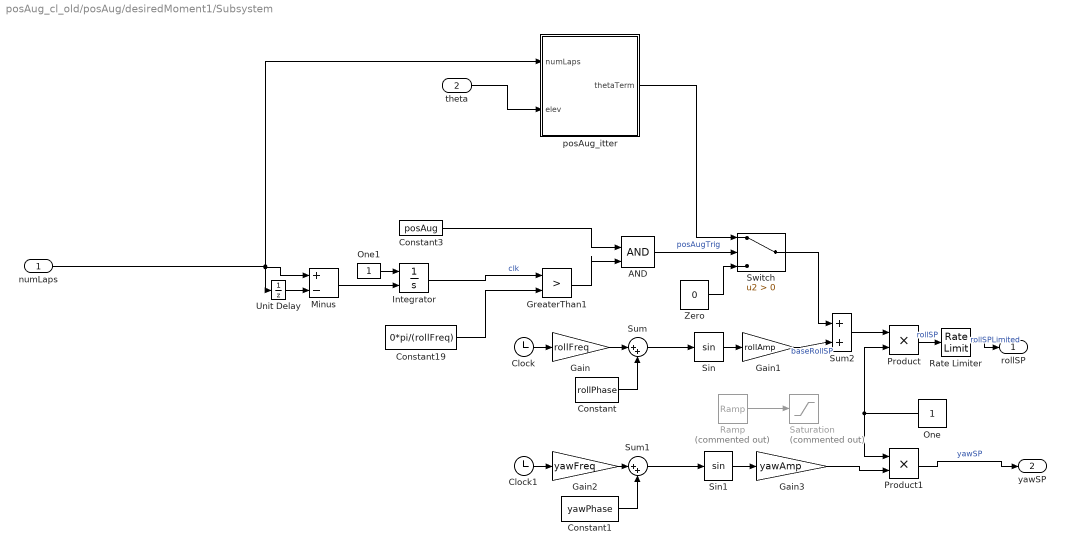
== system posAug_cl_old/posAug/desiredMoment1/Subsystem ==
  numLaps : Inport
  theta : Inport  Port=2
  AND : Logic  IconShape=distinctive  AllPortsSameDT=off  OutDataTypeStr=boolean
  Clock : Clock
  Clock1 : Clock
  Constant : Constant  Value=rollPhase
  Constant1 : Constant  Value=yawPhase
  Constant19 : Constant  Value=0*pi/(rollFreq)
  Constant3 : Constant  Value=posAug
  Gain : Gain  Gain=rollFreq
  Gain1 : Gain  Gain=rollAmp
  Gain2 : Gain  Gain=yawFreq
  Gain3 : Gain  Gain=yawAmp
  GreaterThan1 : RelationalOperator  Operator=>  OutDataTypeStr=boolean  RndMeth=Simplest  InputSameDT=off
  Integrator : Integrator  ExternalReset=rising
  Minus : Sum  Inputs=+-
  One : Constant  OutDataTypeStr=Inherit: Inherit via back propagation
  One1 : Constant  OutDataTypeStr=Inherit: Inherit via back propagation
  Product : Product
  Product1 : Product
  Ramp : simulink/Sources/Ramp  Commented=on  slope=(rollFreq)/(3*2*pi)  start=slfExitTime  InitialOutput=0
  Rate Limiter : RateLimiter  RisingSlewLimit=0.1  FallingSlewLimit=-0.1  SampleTimeMode=inherited
  Saturation : Saturate  Commented=on  UpperLimit=1  LowerLimit=0
  Sin : Trigonometry
  Sin1 : Trigonometry
  Sum : Sum  Inputs=|++
  Sum1 : Sum  Inputs=|++
  Sum2 : Sum  Inputs=|++
  Switch : Switch  Criteria=u2 > Threshold  SaturateOnIntegerOverflow=off  InputSameDT=off
  Unit Delay : UnitDelay  SampleTime=-1  HasFrameUpgradeWarning=on
  Zero : Constant  Value=0  OutDataTypeStr=Inherit: Inherit via back propagation
  posAug_itter : Subsystem
  rollSP : Outport
  yawSP : Outport  Port=2
  wires:
  Clock/1 -> Gain/1
  Gain/1 -> Sum/1
  Sum/1 -> Sin/1
  Constant/1 -> Sum/2
  Sin/1 -> Gain1/1
  Gain1/1 -> Sum2/2  "baseRollSP"
  theta/1 -> posAug_itter/2(elev)
  Gain3/1 -> Product1/2
  Clock1/1 -> Gain2/1
  Sum1/1 -> Sin1/1
  Constant1/1 -> Sum1/2
  Gain2/1 -> Sum1/1
  Sin1/1 -> Gain3/1
  Rate Limiter/1 -> rollSP/1  "rollSPLimited"
  One/1 -> Product/2, Product1/1
  Sum2/1 -> Product/1
  posAug_itter/1(thetaTerm) -> Switch/1
  Zero/1 -> Switch/3
  Switch/1 -> Sum2/1
  Product/1 -> Rate Limiter/1  "rollSP"
  Integrator/1 -> GreaterThan1/1  "clk"
  Constant19/1 -> GreaterThan1/2
  GreaterThan1/1 -> AND/2
  Constant3/1 -> AND/1
  AND/1 -> Switch/2  "posAugTrig"
  numLaps/1 -> Minus/1, Unit Delay/1, posAug_itter/1(numLaps)
  Unit Delay/1 -> Minus/2
  Minus/1 -> Integrator/2
  One1/1 -> Integrator/1
  Ramp/1 -> Saturation/1
  Product1/1 -> yawSP/1  "yawSP"

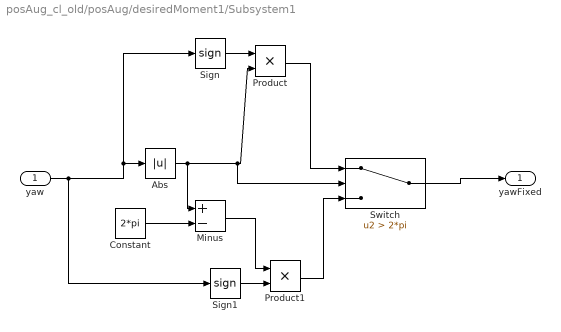
== system posAug_cl_old/posAug/desiredMoment1/Subsystem1 ==
  yaw : Inport
  Abs : Abs  SaturateOnIntegerOverflow=off
  Constant : Constant  Value=2*pi
  Minus : Sum  Inputs=+-
  Product : Product
  Product1 : Product
  Sign : Signum
  Sign1 : Signum
  Switch : Switch  Criteria=u2 > Threshold  Threshold=2*pi  SaturateOnIntegerOverflow=off  InputSameDT=off
  yawFixed : Outport
  wires:
  yaw/1 -> Sign1/1, Abs/1, Sign/1
  Sign/1 -> Product/1
  Abs/1 -> Minus/1, Switch/2, Product/2
  Product/1 -> Switch/1
  Constant/1 -> Minus/2
  Sign1/1 -> Product1/2
  Minus/1 -> Product1/1
  Product1/1 -> Switch/3
  Switch/1 -> yawFixed/1

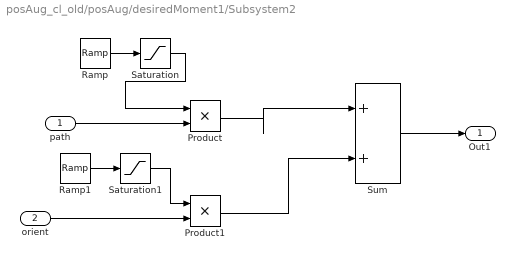
== system posAug_cl_old/posAug/desiredMoment1/Subsystem2 ==
  path : Inport
  orient : Inport  Port=2
  Product : Product
  Product1 : Product
  Ramp : simulink/Sources/Ramp  slope=-1/(2*pi*rollFreq)  start=transTime  InitialOutput=1
  Ramp1 : simulink/Sources/Ramp  slope=1/(2*pi*rollFreq)  start=transTime  InitialOutput=0
  Saturation : Saturate  UpperLimit=1  LowerLimit=0
  Saturation1 : Saturate  UpperLimit=1  LowerLimit=0
  Sum : Sum  Inputs=|++
  Out1 : Outport
  wires:
  Ramp/1 -> Saturation/1
  Saturation/1 -> Product/1
  path/1 -> Product/2
  orient/1 -> Product1/2
  Product/1 -> Sum/1
  Product1/1 -> Sum/2
  Sum/1 -> Out1/1
  Saturation1/1 -> Product1/1
  Ramp1/1 -> Saturation1/1

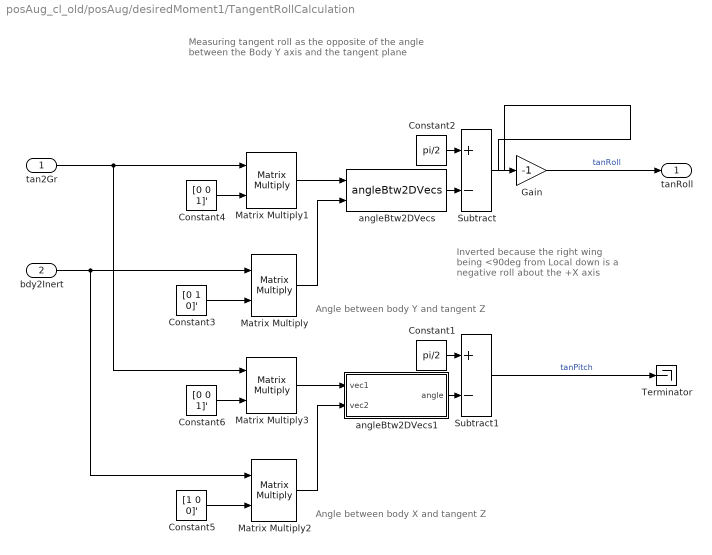
== system posAug_cl_old/posAug/desiredMoment1/TangentRollCalculation ==
  note: Angle between body X and tangent Z
  note: Inverted because the right wing
      | being <90deg from Local down
      | is a negative roll about the +X axis
  note: Angle between body Y and tangent Z
  note: Measuring tangent roll as the opposite
      | of the angle between the Body Y axis
      | and the tangent plane
  tan2Gr : Inport
  bdy2Inert : Inport  Port=2
  Constant1 : Constant  Value=pi/2
  Constant2 : Constant  Value=pi/2
  Constant3 : Constant  Value=[0 1 0]'
  Constant4 : Constant  Value=[0 0 1]'
  Constant5 : Constant  Value=[1 0 0]'
  Constant6 : Constant  Value=[0 0 1]'
  Gain : Gain  Gain=-1
  Matrix Multiply{,1..3} (4 alike) : Product  Multiplication=Matrix(*)
  Subtract : Sum  Inputs=+-
  Subtract1 : Sum  Inputs=+-
  Terminator : Terminator
  angleBtw2DVecs : angleBtw2Vecs_ul/angleBtw2DVecs  SystemSampleTime=-1  VariantActivationTime=update diagram  Latency=0  AutoFrameSizeCalculation=off
  angleBtw2DVecs1 : Subsystem
  tanRoll : Outport  VectorParamsAs1DForOutWhenUnconnected=off
  wires:
  Constant5/1 -> Matrix Multiply2/2
  angleBtw2DVecs1/1(angle) -> Subtract1/2
  Constant1/1 -> Subtract1/1
  Matrix Multiply3/1 -> angleBtw2DVecs1/1(vec1)
  Constant6/1 -> Matrix Multiply3/2
  Matrix Multiply2/1 -> angleBtw2DVecs1/2(vec2)
  tan2Gr/1 -> Matrix Multiply1/1, Matrix Multiply3/1
  Subtract1/1 -> Terminator/1  "tanPitch"
  bdy2Inert/1 -> Matrix Multiply/1, Matrix Multiply2/1
  Gain/1 -> tanRoll/1  "tanRoll"
  Matrix Multiply/1 -> angleBtw2DVecs/2
  Constant4/1 -> Matrix Multiply1/2
  Matrix Multiply1/1 -> angleBtw2DVecs/1
  Constant2/1 -> Subtract/1
  angleBtw2DVecs/1 -> Subtract/2
  Constant3/1 -> Matrix Multiply/2
  Subtract/1 -> Gain/1

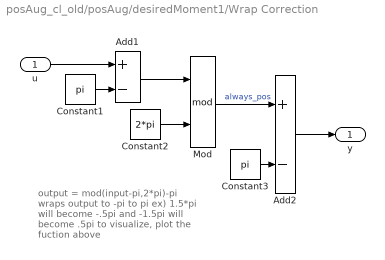
== system posAug_cl_old/posAug/desiredMoment1/Wrap Correction ==
  note: output = mod(input-pi,2*pi)-pi
      | wraps output to -pi to pi
      |
      | ex) 1.5*pi will become -.5pi
      | 	and -1.5pi will become .5pi
      |
      | to visualize, plot the fuction above
  u : Inport
  Add1 : Sum  Inputs=+-
  Add2 : Sum  Inputs=+-
  Constant1 : Constant  Value=pi
  Constant2 : Constant  Value=2*pi
  Constant3 : Constant  Value=pi
  Mod : Math  Operator=mod  SignedPower=on
  y : Outport  VectorParamsAs1DForOutWhenUnconnected=off
  wires:
  Add2/1 -> y/1
  Constant3/1 -> Add2/2
  Mod/1 -> Add2/1  "always_pos"
  Constant2/1 -> Mod/2
  Add1/1 -> Mod/1
  Constant1/1 -> Add1/2
  u/1 -> Add1/1
